simulink model "StSys_TrqShutOff"  (R2016b)
settings: configuration reference "CodeGenConfigSet" (kept outside this file)
values from neighbouring files (symbols this model uses):
  StSys_stTrqShutOff_C = Calibration.Parameter    [init_StSys_TrqShutOff.m]
  StSys_trqSetAdjVal_C = Calibration.Parameter    [init_StSys_TrqShutOff.m]
settings Model: Creator=lenovo  LastModifiedBy=lenovo
settings ConfigSetRef: SourceLocation=Base Workspace

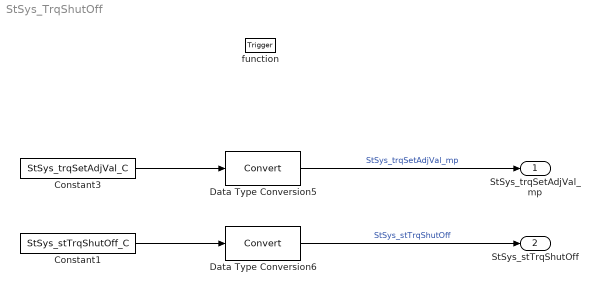
== system StSys_TrqShutOff ==
  function : TriggerPort  TriggerType=function-call  VariantControl=Variant
  Constant1 : Constant  Value=StSys_stTrqShutOff_C
  Constant3 : Constant  Value=StSys_trqSetAdjVal_C
  Data Type Conversion5 : DataTypeConversion
  Data Type Conversion6 : DataTypeConversion
  StSys_trqSetAdjVal_mp : Outport  Tag=Nm  Description=EPPROM adjustment value for start torque correction  OutMin=0  OutMax=1000  OutDataTypeStr=Trq_Nm
  StSys_stTrqShutOff : Outport  Description=the status of the starting torque shuto-off input  Port=2  OutMin=0  OutMax=1  OutDataTypeStr=boolean
  wires:
  Constant3/1 -> Data Type Conversion5/1
  Constant1/1 -> Data Type Conversion6/1
  Data Type Conversion5/1 -> StSys_trqSetAdjVal_mp/1  "StSys_trqSetAdjVal_mp"
  Data Type Conversion6/1 -> StSys_stTrqShutOff/1  "StSys_stTrqShutOff"
